simulink model "BodyModel"  (R2018b)
settings: Solver=VariableStepAuto  StartTime=0.0  StopTime=10  RelTol=1e-3
values from neighbouring files (symbols this model uses):
  a = 1    [Part1_Graphs.m]    (also in SetCoefficients.m = 1.25)
  g = 9.81    [SetCoefficients.m]    (also in SetCoefficients_QC.m)
  m1 = mb/2    (= 250)    [SetCoefficients.m]    (also in SetCoefficients_QC.m)
settings Model: Creator=jtb32  LastModifiedBy=joebe
settings SFSimCC: SimUseLocalCustomCode=off
settings RTWCC: RTWUseLocalCustomCode=off

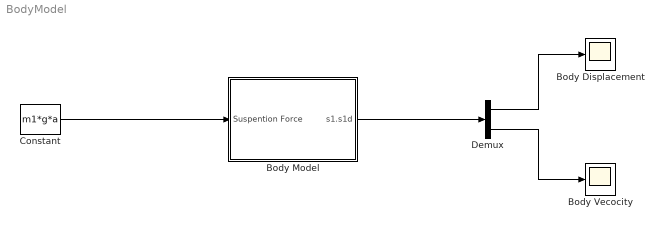
== system BodyModel ==
  Body Displacement : Scope
  Body Model : Subsystem
  Body Vecocity : Scope
  Constant : Constant  Value=m1*g*a
  Demux : Demux  Outputs=2
  wires:
  Body Model/1(s1.s1d) -> Demux/1
  Demux/2 -> Body Vecocity/1
  Demux/1 -> Body Displacement/1
  Constant/1 -> Body Model/1("Suspention Force ")

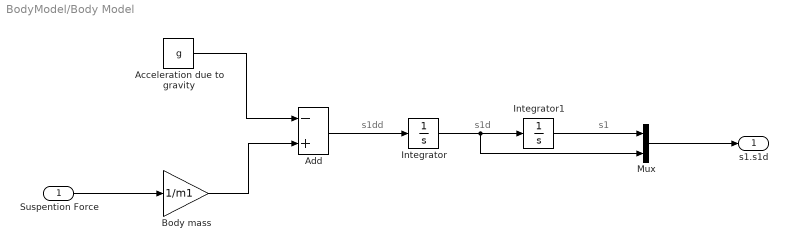
== system BodyModel/Body Model ==
  note: s1d
  note: s1
  note: s1dd
  "Suspention Force " : Inport
  Acceleration due to gravity : Constant  Value=g
  Add : Sum  Inputs=-+
  Body mass : Gain  Gain=1/m1
  Integrator : Integrator
  Integrator1 : Integrator
  Mux : Mux  Inputs=2
  s1.s1d : Outport
  wires:
  Body mass/1 -> Add/2
  Integrator/1 -> Mux/2, Integrator1/1
  Add/1 -> Integrator/1
  Acceleration due to gravity/1 -> Add/1
  Integrator1/1 -> Mux/1
  "Suspention Force "/1 -> Body mass/1
  Mux/1 -> s1.s1d/1
